simulink model "SmartGridFinal"  (R2018a)
settings: Solver=VariableStepAuto  StartTime=0.0  StopTime=10.0  RelTol=1e-3
libraries: powerlib x26, powerlib_meascontrol x7, simulink x5, re_lib x1
settings Model: Creator=Preetham  LastModifiedBy=Preetham

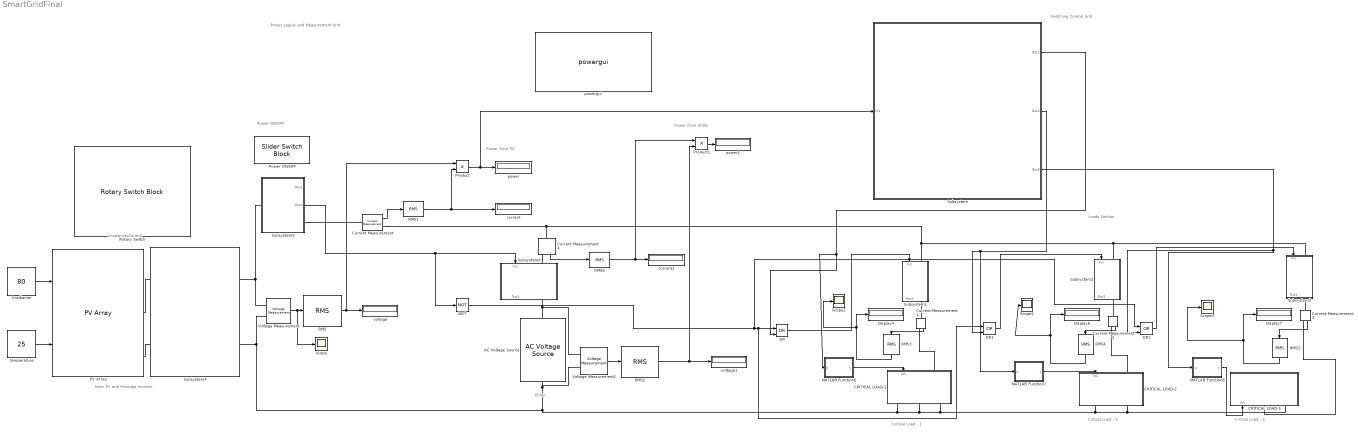
== system SmartGridFinal ==
  note: Power ON/OFF
  note: Utility
  note: Solar PV and H-bridge Inverter
  note: Loads Section
  note: Switching Control Unit
  note: Power supply and Measurement Unit
  note: Power from PV
  note: Power from Utility
  note: Critical Load - 1
  note: Critical Load - 2
  note: Critical Load - 3
  note: Irradiance Control
  AC Voltage Source : powerlib/Electrical Sources/AC Voltage Source  Amplitude=315  Phase=0  Frequency=50  SampleTime=0  Measurements=None  BusType=swing  Pref=10e3  Qref=0  Qmin=-inf  Qmax=+inf
  CRITICAL LOAD-1 : Subsystem
  CRITICAL LOAD-2 : Subsystem
  CRITICAL LOAD-3 : Subsystem
  Current Measurement{,1..4} (5 alike) : powerlib/Measurements/Current Measurement  PhasorSimulation=off  OutputType=Complex  PSBequivalent=0
  Display4 : Display
  Display6 : Display
  Display7 : Display
  Irradiance : Constant  Value=80
  MATLAB Function6 : MATLAB Function  TreatAsAtomicUnit=on
  MATLAB Function7 : MATLAB Function  TreatAsAtomicUnit=on
  "MATLAB Function8 " : MATLAB Function  TreatAsAtomicUnit=on
  NOT : Logic  Operator=NOT  IconShape=distinctive  AllPortsSameDT=off  OutDataTypeStr=boolean
  OR : Logic  Operator=OR  IconShape=distinctive  AllPortsSameDT=off  OutDataTypeStr=boolean
  OR1 : Logic  Operator=OR  IconShape=distinctive  AllPortsSameDT=off  OutDataTypeStr=boolean
  OR2 : Logic  Operator=OR  IconShape=distinctive  AllPortsSameDT=off  OutDataTypeStr=boolean
  PV Array : re_lib/Solar/PV Array  Npar=20  Nser=10  PlotType=array @ 1000 W/m2 & specified temperatures  S_vec="[ 150  80  60 ]"  Temp_C_vec="[ 45 25  ]"  ModuleName=1Soltech 1STH-215-P  PlotWhenSelected=off  Pm=213.15  Ncell=60  Voc=36.3  Isc=7.84  Vm=29  Im=7.35  beta_Voc_pc=-0.36099  alpha_Isc_pc=0.102  beta_Voc=-0.13104  alpha_Isc=0.007997  IL=7.8649  I0=2.9259e-10  nI=0.98117  Rsh=313.3991  Rs=0.39383  BAL=off  Tc=1e-6  Tfilter=5e-5
  Power ON/OFF : SliderSwitchBlock  WebBlockId=143
      settings: Values={{'Off', 'On'}, [1 0]}
  Product : Product
  Product1 : Product
  RMS{,1..6} (7 alike) : powerlib_meascontrol/Measurements/RMS  TrueRMS=on  Freq=60  RMSInit=120  Ts=0
  Rotary Switch : RotarySwitchBlock  WebBlockId=257
      settings: Values={{'Low Irradiance', 'Medium Irradiance', 'High Irradiance'}, [40 80 150]}
  Scope{,1..3} (4 alike) : Scope
  Subsystem : Subsystem
  Subsystem1 : Subsystem
  Subsystem2 : Subsystem
  Subsystem3 : Subsystem
  Subsystem4 : Subsystem
  Subsystem5 : Subsystem
  Subsystem6 : Subsystem
  Voltage Measurement : powerlib/Measurements/Voltage Measurement  PhasorSimulation=off  OutputType=Complex  PSBequivalent=0
  Voltage Measurement1 : powerlib/Measurements/Voltage Measurement  PhasorSimulation=off  OutputType=Complex  PSBequivalent=0
  current : Display
  current1 : Display
  power : Display
  power1 : Display
  powergui : powerlib/powergui  Priority=1  SimulationMode=Continuous  SampleTime=50e-6  frequency=60  Iterations=50  frequencyindice=0  Pbase=100e6  ErrMax=1e-4  UnitsV=kV  UnitsW=MW  buscounter=0  FunctionMessages=off  echomessages=off  EnableUseOfTLC=off  CurrentSourceSwitches=off  DisableSnubberDevices=off  DisableRonSwitches=off  DisableVfSwitches=off  DisplayEquations=off  SolverType=Tustin/Backward Euler (TBE)  Interpol=off  ExternalGateDelay=off  methode=off  Ts=100  x0status=blocks  SPID=on  SwTol=0  HookPort=off  RestoreLinks=warning  ResistiveCurrentMeasurement=off  Frange=[0:2:500]  Ylog=off  Xlog=on  ShowGrid=off  save=off  variable=ZData  structure=0  ZoomFFT=off  StartTime=0.0  cycles=1  DisplayStyle=1  fundamental=60  FreqAxis=off  MaxFrequency=1000  frequencyindicesteady=1  RmsSteady=1  display=off
  temperature : Constant  Value=25
  voltage : Display
  voltage1 : Display
  wires:
  Product1/1 -> power1/1
  Subsystem5/2(Out2) -> NOT/1, Subsystem6/1(In1)
  RMS6/1 -> Product1/1, current1/1
  Current Measurement4/1 -> RMS6/1
  Product/1 -> Subsystem/1(In1), power/1
  Subsystem/3(Out3) -> "MATLAB Function8 "/1(u), OR2/2
  "MATLAB Function8 "/1(y) -> CRITICAL LOAD-3/1(In1)
  MATLAB Function7/1(y) -> CRITICAL LOAD-2/1(In1)
  RMS5/1 -> Scope3/1, Display7/1
  Current Measurement1/1 -> RMS3/1
  RMS4/1 -> Scope2/1, Display6/1
  Irradiance/1 -> PV Array/1
  RMS3/1 -> Scope1/1, Display4/1
  RMS/1 -> voltage/1, Product/1
  Subsystem/1(Out1) -> OR/2, MATLAB Function6/1(u)
  Current Measurement2/1 -> RMS4/1
  temperature/1 -> PV Array/2
  RMS1/1 -> Product/2, current/1
  MATLAB Function6/1(y) -> CRITICAL LOAD-1/1(In1)
  Subsystem/2(Out2) -> OR1/2, MATLAB Function7/1(u)
  Voltage Measurement/1 -> Scope/1, RMS/1
  Current Measurement3/1 -> RMS5/1
  RMS2/1 -> Product1/2, voltage1/1
  Voltage Measurement1/1 -> RMS2/1
  Current Measurement/1 -> RMS1/1
  OR/1 -> Subsystem1/1(In1)
  OR1/1 -> Subsystem2/1(In1)
  OR2/1 -> Subsystem3/1(In1)
  NOT/1 -> OR1/1, OR/1, OR2/1
  connections:
  CRITICAL LOAD-1/RConn1 -- CRITICAL LOAD-1/RConn2 -- CRITICAL LOAD-1/RConn3 -- CRITICAL LOAD-2/RConn1 -- CRITICAL LOAD-3/LConn2 -- CRITICAL LOAD-2/RConn2 -- Voltage Measurement1/LConn2 -- AC Voltage Source/LConn1 -- Voltage Measurement/LConn2 -- Subsystem4/RConn2
  Subsystem4/RConn1 -- Subsystem5/LConn1 -- Voltage Measurement/LConn1
  Subsystem3/LConn1 -- Current Measurement/RConn1 -- Current Measurement4/LConn1 -- Subsystem1/LConn1 -- Subsystem2/LConn1
  Voltage Measurement1/LConn1 -- Subsystem6/RConn1 -- AC Voltage Source/RConn1
  Subsystem5/RConn1 -- Current Measurement/LConn1
  Current Measurement2/RConn1 -- CRITICAL LOAD-2/LConn1
  Current Measurement4/RConn1 -- Subsystem6/LConn1
  Current Measurement2/LConn1 -- Subsystem2/RConn1
  Current Measurement3/LConn1 -- Subsystem3/RConn1
  Subsystem4/LConn1 -- PV Array/RConn1
  Subsystem4/LConn2 -- PV Array/RConn2
  Current Measurement1/RConn1 -- CRITICAL LOAD-1/LConn1
  Subsystem1/RConn1 -- Current Measurement1/LConn1
  Current Measurement3/RConn1 -- CRITICAL LOAD-3/LConn1

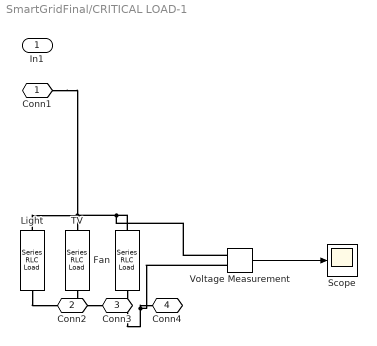
== system SmartGridFinal/CRITICAL LOAD-1 ==
  In1 : Inport
  Fan : powerlib/Elements/Series RLC Load  LConnTagsString=a  RConnTagsString=__new0  NominalVoltage=220  NominalFrequency=50  ActivePower=25  InductivePower=0  CapacitivePower=0  Setx0=off  InitialVoltage=0  SetiL0=off  InitialCurrent=0  Measurements=None  LoadType=constant Z
  Light : powerlib/Elements/Series RLC Load  LConnTagsString=a  RConnTagsString=__new0  NominalVoltage=220  NominalFrequency=50  ActivePower=40  InductivePower=0  CapacitivePower=0  Setx0=off  InitialVoltage=0  SetiL0=off  InitialCurrent=0  Measurements=None  LoadType=constant Z
  Scope : Scope
  TV : powerlib/Elements/Series RLC Load  LConnTagsString=a  RConnTagsString=__new0  NominalVoltage=220  NominalFrequency=50  ActivePower=120  InductivePower=0  CapacitivePower=0  Setx0=off  InitialVoltage=0  SetiL0=off  InitialCurrent=0  Measurements=None  LoadType=constant Z
  Voltage Measurement : powerlib/Measurements/Voltage Measurement  PhasorSimulation=off  OutputType=Complex  PSBequivalent=0
  Conn1 : PMIOPort  Side=Left
  Conn2 : PMIOPort  Port=2  Side=Right
  Conn3 : PMIOPort  Port=3  Side=Right
  Conn4 : PMIOPort  Port=4  Side=Right
  wires:
  Voltage Measurement/1 -> Scope/1
  connections:
  Light/LConn1 -- Voltage Measurement/LConn1 -- Fan/LConn1 -- Conn1/RConn1 -- TV/LConn1
  Light/RConn1 -- Conn2/RConn1
  TV/RConn1 -- Conn3/RConn1
  Fan/RConn1 -- Voltage Measurement/LConn2 -- Conn4/RConn1

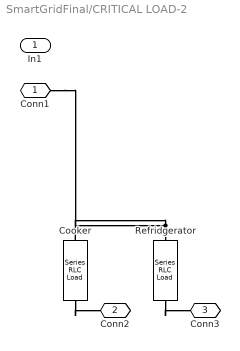
== system SmartGridFinal/CRITICAL LOAD-2 ==
  In1 : Inport
  Cooker : powerlib/Elements/Series RLC Load  LConnTagsString=a  RConnTagsString=__new0  NominalVoltage=220  NominalFrequency=50  ActivePower=1100  InductivePower=0  CapacitivePower=0  Setx0=off  InitialVoltage=0  SetiL0=off  InitialCurrent=0  Measurements=None  LoadType=constant Z
  Refridgerator : powerlib/Elements/Series RLC Load  LConnTagsString=a  RConnTagsString=__new0  NominalVoltage=220  NominalFrequency=50  ActivePower=500  InductivePower=0  CapacitivePower=0  Setx0=off  InitialVoltage=0  SetiL0=off  InitialCurrent=0  Measurements=None  LoadType=constant Z
  Conn1 : PMIOPort  Side=Left
  Conn2 : PMIOPort  Port=2  Side=Right
  Conn3 : PMIOPort  Port=3  Side=Right
  connections:
  Refridgerator/LConn1 -- Conn1/RConn1 -- Cooker/LConn1
  Cooker/RConn1 -- Conn2/RConn1
  Refridgerator/RConn1 -- Conn3/RConn1

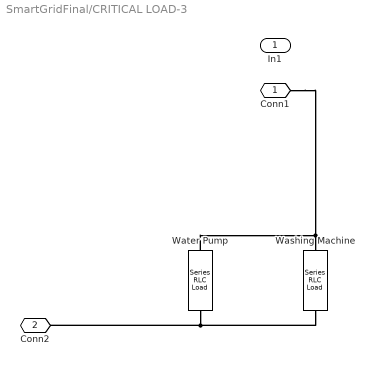
== system SmartGridFinal/CRITICAL LOAD-3 ==
  In1 : Inport
  Washing Machine : powerlib/Elements/Series RLC Load  LConnTagsString=a  RConnTagsString=__new0  NominalVoltage=220  NominalFrequency=50  ActivePower=500  InductivePower=0  CapacitivePower=0  Setx0=off  InitialVoltage=0  SetiL0=off  InitialCurrent=0  Measurements=None  LoadType=constant Z
  Water Pump : powerlib/Elements/Series RLC Load  LConnTagsString=a  RConnTagsString=__new0  NominalVoltage=220  NominalFrequency=50  ActivePower=1800  InductivePower=0  CapacitivePower=0  Setx0=off  InitialVoltage=0  SetiL0=off  InitialCurrent=0  Measurements=None  LoadType=constant Z
  Conn1 : PMIOPort  Side=Left
  Conn2 : PMIOPort  Port=2  Side=Left
  connections:
  Water Pump/RConn1 -- Conn2/RConn1 -- Washing Machine/RConn1
  Washing Machine/LConn1 -- Conn1/RConn1 -- Water Pump/LConn1

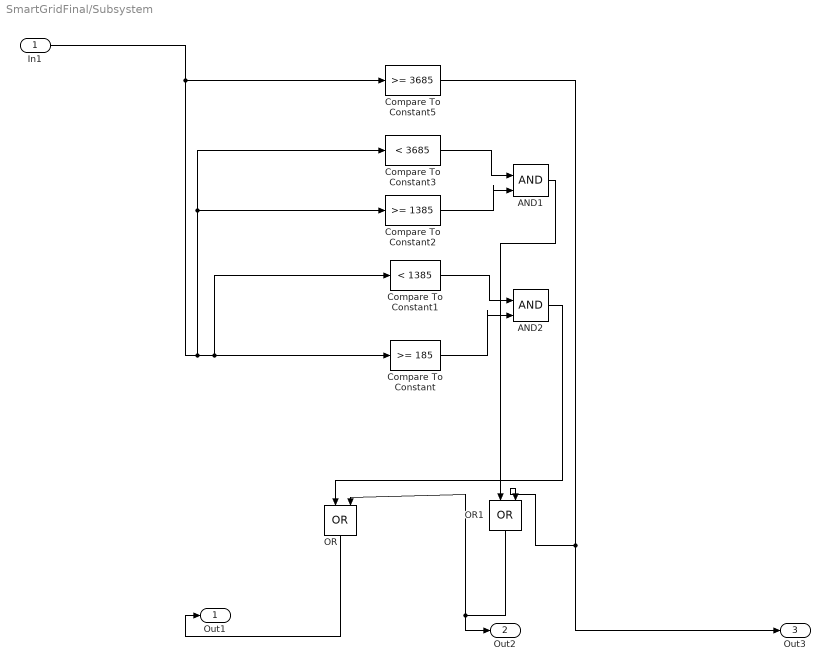
== system SmartGridFinal/Subsystem ==
  In1 : Inport
  AND1 : Logic  IconShape=distinctive  AllPortsSameDT=off  OutDataTypeStr=boolean
  AND2 : Logic  IconShape=distinctive  AllPortsSameDT=off  OutDataTypeStr=boolean
  Compare To Constant : simulink/Logic and Bit Operations/Compare To Constant  relop=>=  const=185  OutDataTypeStr=boolean
  Compare To Constant1 : simulink/Logic and Bit Operations/Compare To Constant  relop=<  const=1385  OutDataTypeStr=boolean
  Compare To Constant2 : simulink/Logic and Bit Operations/Compare To Constant  relop=>=  const=1385  OutDataTypeStr=boolean
  Compare To Constant3 : simulink/Logic and Bit Operations/Compare To Constant  relop=<  const=3685  OutDataTypeStr=boolean
  Compare To Constant5 : simulink/Logic and Bit Operations/Compare To Constant  relop=>=  const=3685  OutDataTypeStr=boolean
  OR : Logic  Operator=OR  IconShape=distinctive  AllPortsSameDT=off  OutDataTypeStr=boolean
  OR1 : Logic  Operator=OR  IconShape=distinctive  AllPortsSameDT=off  OutDataTypeStr=boolean
  Out1 : Outport
  Out2 : Outport  Port=2
  Out3 : Outport  Port=3
  wires:
  AND1/1 -> OR1/1
  In1/1 -> Compare To Constant1/1, Compare To Constant/1, Compare To Constant2/1, Compare To Constant3/1, Compare To Constant5/1
  Compare To Constant1/1 -> AND2/1
  Compare To Constant2/1 -> AND1/2
  AND2/1 -> OR/1
  Compare To Constant/1 -> AND2/2
  Compare To Constant3/1 -> AND1/1
  Compare To Constant5/1 -> Out3/1, OR1/2
  OR1/1 -> Out2/1, OR/2
  OR/1 -> Out1/1

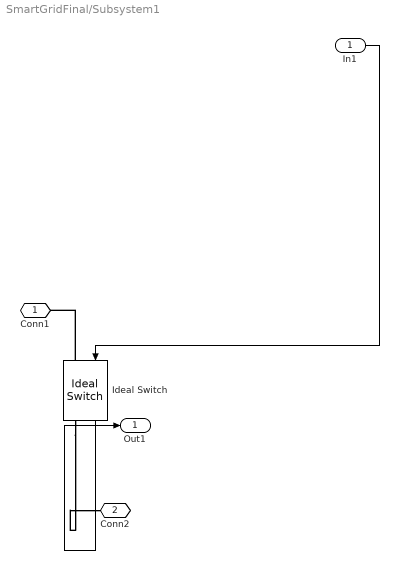
== system SmartGridFinal/Subsystem1 ==
  In1 : Inport
  Ideal Switch : powerlib/Power Electronics/Ideal Switch  Ron=0.001  Lon=0  IC=0  Rs=1e5  Cs=inf  Measurements=on
  Conn1 : PMIOPort  Side=Left
  Conn2 : PMIOPort  Port=2  Side=Right
  Out1 : Outport
  wires:
  In1/1 -> Ideal Switch/1
  Ideal Switch/1 -> Out1/1
  connections:
  Ideal Switch/RConn1 -- Conn2/RConn1
  Ideal Switch/LConn1 -- Conn1/RConn1

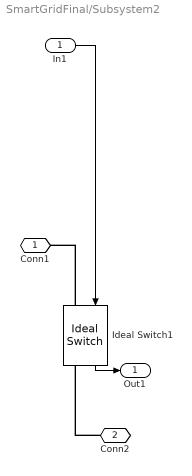
== system SmartGridFinal/Subsystem2 ==
  In1 : Inport
  Ideal Switch1 : powerlib/Power Electronics/Ideal Switch  Ron=0.001  Lon=0  IC=0  Rs=1e5  Cs=inf  Measurements=on
  Conn1 : PMIOPort  Side=Left
  Conn2 : PMIOPort  Port=2  Side=Right
  Out1 : Outport
  wires:
  In1/1 -> Ideal Switch1/1
  Ideal Switch1/1 -> Out1/1
  connections:
  Conn2/RConn1 -- Ideal Switch1/RConn1
  Ideal Switch1/LConn1 -- Conn1/RConn1

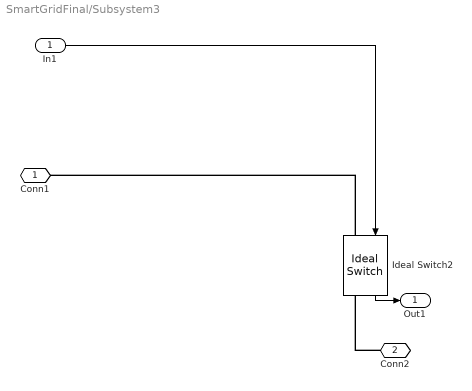
== system SmartGridFinal/Subsystem3 ==
  In1 : Inport
  Ideal Switch2 : powerlib/Power Electronics/Ideal Switch  Ron=0.001  Lon=0  IC=0  Rs=1e5  Cs=inf  Measurements=on
  Conn1 : PMIOPort  Side=Left
  Conn2 : PMIOPort  Port=2  Side=Right
  Out1 : Outport
  wires:
  In1/1 -> Ideal Switch2/1
  Ideal Switch2/1 -> Out1/1
  connections:
  Ideal Switch2/LConn1 -- Conn1/RConn1
  Conn2/RConn1 -- Ideal Switch2/RConn1

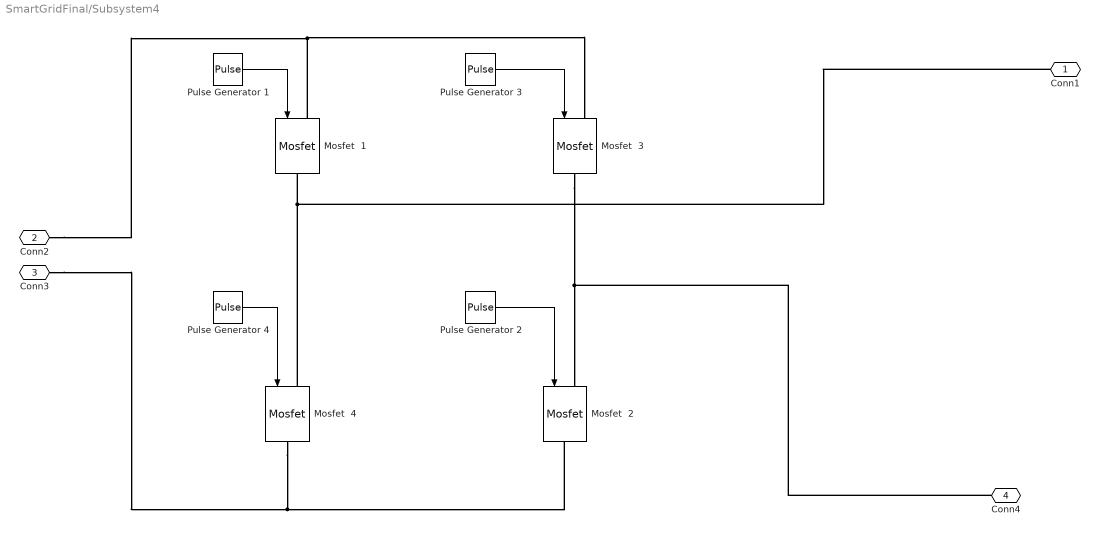
== system SmartGridFinal/Subsystem4 ==
  Mosfet  {1..4} (4 alike) : powerlib/Power Electronics/Mosfet  Ron=0.1  Lon=0  Rd=0.01  Vfd=0  IC=0  Rs=1e5  Cs=inf  Measurements=off
  Pulse Generator 1 : DiscretePulseGenerator  PulseType=Time based  Period=0.02  PulseWidth=50
  Pulse Generator 2 : DiscretePulseGenerator  PulseType=Time based  Period=0.02  PulseWidth=50
  Pulse Generator 3 : DiscretePulseGenerator  PulseType=Time based  Period=0.02  PulseWidth=50  PhaseDelay=0.01
  Pulse Generator 4 : DiscretePulseGenerator  PulseType=Time based  Period=0.02  PulseWidth=50  PhaseDelay=0.01
  Conn1 : PMIOPort  Side=Right
  Conn2 : PMIOPort  Port=2  Side=Left
  Conn3 : PMIOPort  Port=3  Side=Left
  Conn4 : PMIOPort  Port=4  Side=Right
  wires:
  Pulse Generator 3/1 -> Mosfet  3/1
  Pulse Generator 1/1 -> Mosfet  1/1
  Pulse Generator 2/1 -> Mosfet  2/1
  Pulse Generator 4/1 -> Mosfet  4/1
  connections:
  Mosfet  4/LConn1 -- Conn1/RConn1 -- Mosfet  1/RConn1
  Mosfet  3/RConn1 -- Conn4/RConn1 -- Mosfet  2/LConn1
  Mosfet  2/RConn1 -- Conn3/RConn1 -- Mosfet  4/RConn1
  Mosfet  1/LConn1 -- Conn2/RConn1 -- Mosfet  3/LConn1

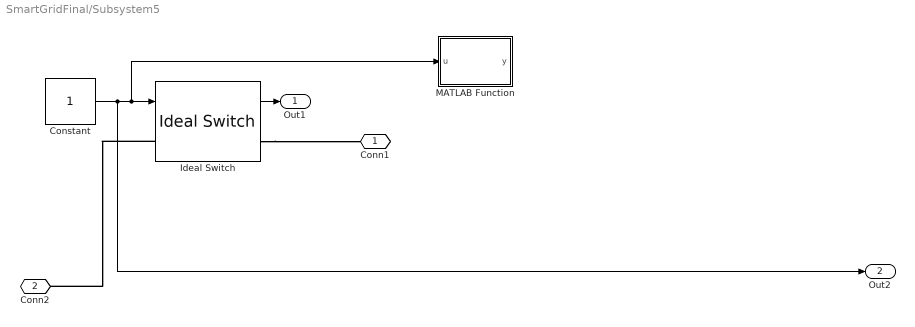
== system SmartGridFinal/Subsystem5 ==
  Constant : Constant
  Ideal Switch : powerlib/Power Electronics/Ideal Switch  Ron=0.001  Lon=0  IC=1  Rs=1e5  Cs=inf  Measurements=on
  MATLAB Function : MATLAB Function  TreatAsAtomicUnit=on
  Conn1 : PMIOPort  Side=Right
  Conn2 : PMIOPort  Port=2  Side=Left
  Out1 : Outport
  Out2 : Outport  Port=2
  wires:
  Ideal Switch/1 -> Out1/1
  Constant/1 -> Out2/1, MATLAB Function/1(u), Ideal Switch/1
  connections:
  Ideal Switch/RConn1 -- Conn1/RConn1
  Ideal Switch/LConn1 -- Conn2/RConn1

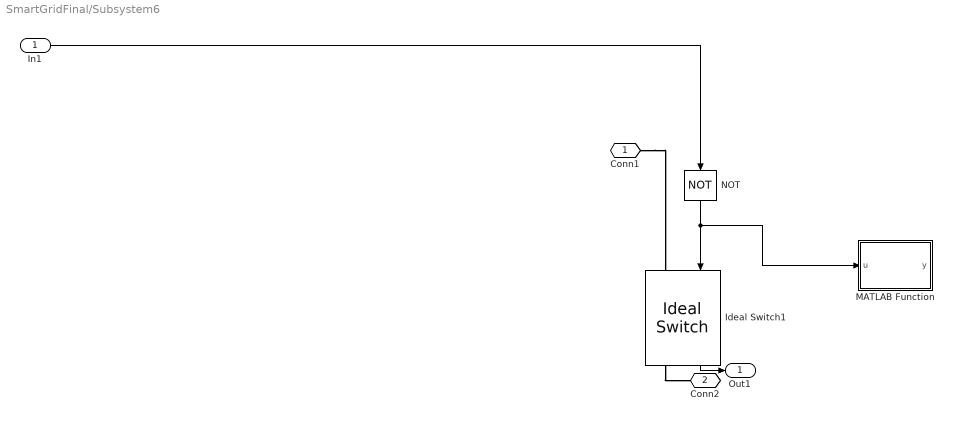
== system SmartGridFinal/Subsystem6 ==
  In1 : Inport
  Ideal Switch1 : powerlib/Power Electronics/Ideal Switch  Ron=0.001  Lon=0  IC=1  Rs=1e5  Cs=inf  Measurements=on
  MATLAB Function : MATLAB Function  TreatAsAtomicUnit=on
  NOT : Logic  Operator=NOT  IconShape=distinctive  AllPortsSameDT=off  OutDataTypeStr=boolean
  Conn1 : PMIOPort  Side=Left
  Conn2 : PMIOPort  Port=2  Side=Right
  Out1 : Outport
  wires:
  Ideal Switch1/1 -> Out1/1
  In1/1 -> NOT/1
  NOT/1 -> MATLAB Function/1(u), Ideal Switch1/1
  connections:
  Ideal Switch1/RConn1 -- Conn2/RConn1
  Conn1/RConn1 -- Ideal Switch1/LConn1

== matlab function SmartGridFinal/MATLAB Function7 ==
  data: u input; y output
function y = recolor(u)
coder.extrinsic('set_param');
if u == 1 
    set_param('SmartGridFinal/CRITICAL LOAD-1','BackgroundColor','green');
    set_param('SmartGridFinal/CRITICAL LOAD-2','BackgroundColor','green');
    set_param('SmartGridFinal/CRITICAL LOAD-3','BackgroundColor','red');
else
end
y = u;

== matlab function SmartGridFinal/MATLAB Function6 ==
  data: u input; y output
function y = recolor(u)
coder.extrinsic('set_param');
if u == 1 
    set_param('SmartGridFinal/CRITICAL LOAD-1','BackgroundColor','green');
    set_param('SmartGridFinal/CRITICAL LOAD-2','BackgroundColor','red');
    set_param('SmartGridFinal/CRITICAL LOAD-3','BackgroundColor','red');
else
end
y = u;

== matlab function SmartGridFinal/MATLAB Function8  ==
  data: u input; y output
function y = recolor(u)
coder.extrinsic('set_param');
if u == 1 
    set_param('SmartGridFinal/CRITICAL LOAD-1','BackgroundColor','green');
    set_param('SmartGridFinal/CRITICAL LOAD-2','BackgroundColor','green');
    set_param('SmartGridFinal/CRITICAL LOAD-3','BackgroundColor','green');
else
end
y = u;

== matlab function SmartGridFinal/Subsystem6/MATLAB Function ==
  data: u input; y output
function y = recolor(u)
coder.extrinsic('set_param');
if u == 1 
    set_param('SmartGridFinal/AC Voltage Source','BackgroundColor','green');
    set_param('SmartGridFinal/Subsystem6','BackgroundColor','green');
else
    set_param('SmartGridFinal/AC Voltage Source','BackgroundColor','red');
    set_param('SmartGridFinal/Subsystem6','BackgroundColor','red');
end
y = u;

== matlab function SmartGridFinal/Subsystem5/MATLAB Function ==
  data: u input; y output
function y = recolor(u)
coder.extrinsic('set_param');
if u == 1 
    set_param('SmartGridFinal/Subsystem4','BackgroundColor','green');
    set_param('SmartGridFinal/Subsystem5','BackgroundColor','green');
else
    set_param('SmartGridFinal/Subsystem4','BackgroundColor','red');
    set_param('SmartGridFinal/Subsystem5','BackgroundColor','red');
end
y = u;
